simulink model "SizeDataCenterCoolingSystem"  (R2025b)
settings: Solver=daessc  StartTime=0.0  StopTime=31449600% hours ~ 8736  MaxStep=3600  RelTol=1e-3  AbsTol=1e-3
PreLoadFcn:
  | if ~exist("modelData")
  |     defaultGeographicalCoordinates;
  | end
undefined symbols (not defined in the file or in its folder): day, DiscIntNeverNeededParam, hour, modelData, month, value, year
libraries: fl_lib x63, nesl_utility x14, buildingEnergy_lib x13, datacenter_lib x5, simulink_extras x3, slpidlib x1
(part 1 of 2)
Description:
  | Data Center Cooling System Design and PUE Analysis
settings Model: Creator=vikrants  LastModifiedBy=vikrants
settings SolverCC: AutoScaleAbsTol=off  AlgebraicLoopSolver=TrustRegion  MaxZcPerStep=1.0
settings DataIOCC: SaveOutput=off  DSMLogging=off  SaveTime=off  ReturnWorkspaceOutputs=off  SignalLoggingName=logsout_SizeDataCenterCoolingSystem
settings DebuggingCC: UnconnectedInputMsg=warning  UnconnectedOutputMsg=warning  UnconnectedLineMsg=warning  SymbolicDimsDataTypeCodeGenerationDiagnostic=none
settings ModelReferenceCC: EnableRefExpFcnMdlSchedulingChecks=on
settings SFSimCC: CustomCodeUndefinedFunction=UseInterfaceOnly
settings RTWCC: GPUComputeCapability=3.5  DLArmComputeVersion=19.05
settings SimscapeCC: SimscapeLogName=simlog_DataCenterEnergyRequirement  SimscapeLogLimitData=off  SimscapeLogDataHistory=10000.0  SimscapeCompileArtifactsDiskCache=on

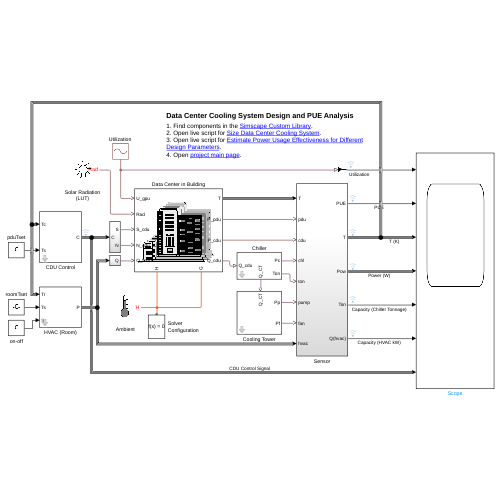
[thumbnail: Simulink's stored preview of the top-level diagram]
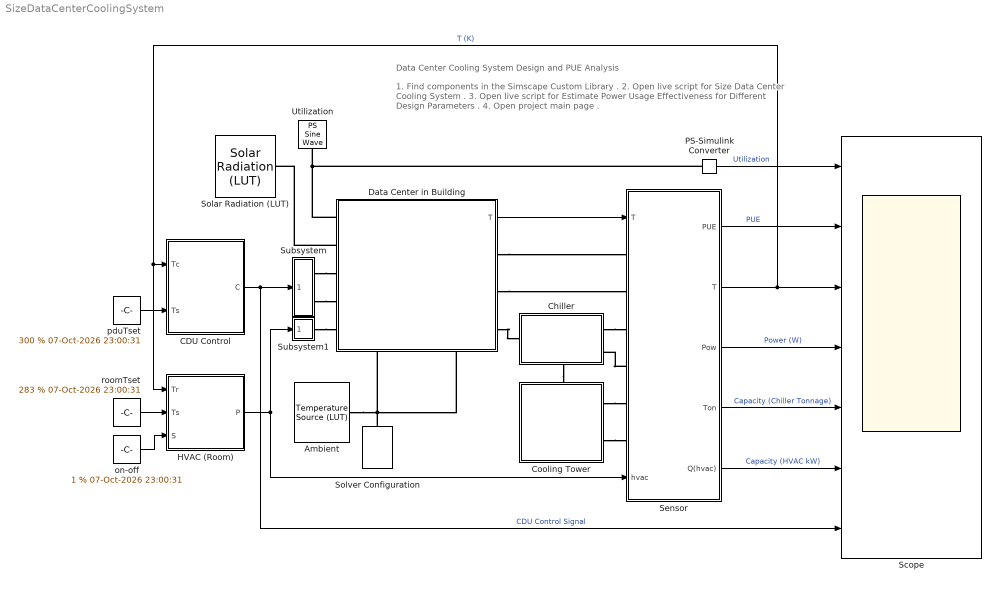
== system SizeDataCenterCoolingSystem ==
  note: 1. Find components in the Simscape Custom Library .
      | 2. Open live script for Size Data Center Cooling System .
      | 3. Open live script for Estimate Power Usage Effectiveness for Different Design Parameters .
      | 4. Open project main page .
  note: Data Center Cooling System Design and PUE Analysis
  Ambient : buildingEnergy_lib/Temperature Source (LUT)  latitude=modelData.Place.Latitude  longitude=modelData.Place.Longitude  localTime=modelData.Place.Meredian  dayLightS=0  startYear=year(modelData.StartDate)  startMonth=month(modelData.StartDate)  startDay=day(modelData.StartDate)  startHr=hour(modelData.StartDate)  numDaysData=ceil(length(modelData.DateTimeVec)/24)  interp_method=simscape.enum.interpolation.linear  extrap_method=simscape.enum.extrapolation.nearest  avgDayTvec="value(modelData.AvgDayT,\"K\") K"  pcDayTvar=modelData.AvgDayTvar  avgNightTvec="value(modelData.AvgNightT,\"K\") K"  pcNightTvar=modelData.AvgNightTvar
      settings: InternalSimscapePortConfiguration="{\"Bottom\":[],\"Left\":[],\"Right\":[{\"id\":\"H\",\"label\":\"H\",\"type\":\"foundation.thermal.thermal\"}],\"Top\":[]}"
  CDU Control : Subsystem  mask{deltaK=50, nPumps=2, tLag=1, motorSpeed=0.01, pidP=100, pidI=10, pidD=1}
      mask prompts: deltaK "Temperature window for no pumping (K)"; nPumps "Number of CDU pumps (-)"; tLag "Measurement time lag (s)"; motorSpeed "Minimum speed ratio of pump motor, 0-1 (-)"; pidP "PID controller P value"; pidI "PID controller I value"; pidD "PID controller D value"
      mask DialogControl Container2 Prompt: Measurements
      mask DialogControl Container3 Prompt: Control
  Chiller : Subsystem  mask{COP=4 % 07-Oct-2026 23:00:31}
      mask prompts: COP "COP (-)"
      settings: PortSchema="{\"entries\":[{\"content\":{\"sides\":[{\"content\":{\"connectorIds\":[\"LConn1\"]},\"type\":\"ConnectorPlacement.EquallySpacedRectSide\",\"uuid\":\"7a9d3cbb-7ec7-4e9b-b3ea-286c7e3ae193\"},{\"content\":{\"connectorIds\":[\"RConn1\",\"RConn2\"],\"side\":\"RIGHT\"},\"type\":\"ConnectorPlacement.EquallySpacedRectSide\",\"uuid\":\"cbc58f31-b5f2-4c0a-b506-28ee5b0234c2\"},{\"content\":{\"side\":\"TOP\"},\"type\":\"ConnectorPlacement.EquallySpacedRectSide\",\"uuid\":\"952b37a4-b854-4a7b-ada4-56afc544f2f3\"},{\"content\":{\"connectorIds\":[\"RConn3\"],\"side\":\"BOTTOM\"},\"type\":\"ConnectorPlacement.EquallySpacedRectSide\",\"uuid\":\"8b8e3134-7703-4e08-8e7e-92d58577d9f6\"}]},\"type\":\"ConnectorPlacement.EquallySpacedConnector\",\"uuid\":\"7e6274f1-c7d7-4742-a570-a83c5958005a\"}],\"packageUris\":[\"http://schema.mathworks.com/mf0/Connector/R2020b\"],\"version\":\"1.0\"}"
      mask DialogControl Container2 Prompt: Chiller Specifications
  Cooling Tower : Subsystem  mask{pumpHead=50, pumpEff=80 % 07-Oct-2026 23:00:31, twrFanRatio=0.02 % 07-Oct-2026 23:00:31, twrRangeDT=8 % 07-Oct-2026 23:00:31}
      mask prompts: pumpHead "Pump nominal head (m)"; pumpEff "Efficiency (%)"; twrFanRatio "Tower fan power ratio (-)"; twrRangeDT "Tower temperature range (degC)"
      settings: PortSchema="{\"entries\":[{\"content\":{\"sides\":[{\"content\":{},\"type\":\"ConnectorPlacement.EquallySpacedRectSide\",\"uuid\":\"457aae9f-8f1f-47f0-962c-a70f6cd1f469\"},{\"content\":{\"connectorIds\":[\"RConn1\",\"RConn2\"],\"side\":\"RIGHT\"},\"type\":\"ConnectorPlacement.EquallySpacedRectSide\",\"uuid\":\"5bf1e4a2-0663-4efc-92dd-183324f83000\"},{\"content\":{\"connectorIds\":[\"LConn1\"],\"side\":\"TOP\"},\"type\":\"ConnectorPlacement.EquallySpacedRectSide\",\"uuid\":\"d9f2a691-48b9-4171-b6ac-f2f0a72efb10\"}]},\"type\":\"ConnectorPlacement.EquallySpacedConnector\",\"uuid\":\"2c0f61f0-4d62-4861-80e7-d1979f22a216\"}],\"packageUris\":[\"http://schema.mathworks.com/mf0/Connector/R2020b\"],\"version\":\"1.0\"}"
      mask DialogControl Container2 Prompt: Pump
      mask DialogControl Container3 Prompt: Cooling Tower
  Data Center in Building : Subsystem
      settings: PortSchema="{\"entries\":[{\"content\":{\"sides\":[{\"content\":{\"connectorIds\":[\"LConn1\",\"LConn2\",\"LConn3\",\"LConn4\",\"LConn5\"]},\"type\":\"ConnectorPlacement.EquallySpacedRectSide\",\"uuid\":\"bcc62a9a-507d-448c-9844-f501869a29d6\"},{\"content\":{\"connectorIds\":[\"Out1\",\"RConn1\",\"RConn2\",\"RConn3\"],\"side\":\"RIGHT\"},\"type\":\"ConnectorPlacement.EquallySpacedRectSide\",\"uuid\":\"b7eb240b-2350-4e54-8431-6517b7627c9e\"},{\"content\":{\"side\":\"TOP\"},\"type\":\"ConnectorPlacement.EquallySpacedRectSide\",\"uuid\":\"331ce5d5-58db-415f-985d-83ca136d8ad7\"},{\"content\":{\"connectorIds\":[\"RConn4\",\"RConn5\"],\"side\":\"BOTTOM\"},\"type\":\"ConnectorPlacement.EquallySpacedRectSide\",\"uuid\":\"0b365461-c329-434a-a979-456a33a1343a\"}]},\"type\":\"ConnectorPlacement.EquallySpacedConnector\",\"uuid\":\"6bcf5050-5add-4254-8764-d57ae143c511\"}],\"packageUris\":[\"http://schema.mathworks.com/mf0/Connector/R2020b\"],\"version\":\"1.0\"}"
      mask Display: image('datacenterLibIcon.png');
  HVAC (Room) : Subsystem  mask{effHeatExchanger=78 % 07-Oct-2026 23:00:31, tLag=1, roomLen=100 % 07-Oct-2026 23:00:31, roomWid=40 % 07-Oct-2026 23:00:31, roomHt=5 % 07-Oct-2026 23:00:31, fracRoomVolDC=0.8 % 07-Oct-2026 23:00:31}
      mask prompts: effHeatExchanger "Efficiency (%)"; tLag "Measurement delay (s)"; roomLen "Length (m)"; roomWid "Width (m)"; roomHt "Height (m)"; fracRoomVolDC "Fraction of room volume occupied by data center (-)"
      mask DialogControl Container3 Prompt: Heat Exchanger
      mask DialogControl Container2 Prompt: Room Details
  PS-Simulink Converter : nesl_utility/PS-Simulink Converter  PhysicalDomain=network_engine_domain  SubClassName=ps_output  LeftPortType=input  RightPortType=output  PseudoPeriodic=off  Frequencies=[]  VectorFormat=inherit  Unit=inherit  AffineConversion=off
  Scope : Scope  NumInputPorts=7
      settings: ActiveDisplayYMinimum=-0.11249999999999996  ActiveDisplayYMaximum=1.1125
  Sensor : Subsystem
      settings: PortSchema="{\"entries\":[{\"content\":{\"sides\":[{\"content\":{\"connectorIds\":[\"In1\",\"LConn1\",\"LConn2\",\"LConn3\",\"LConn4\",\"LConn5\",\"LConn6\",\"In2\"]},\"type\":\"ConnectorPlacement.EquallySpacedRectSide\",\"uuid\":\"a061da3e-4dcb-442c-95d1-d8c22b8cd076\"},{\"content\":{\"connectorIds\":[\"Out1\",\"Out2\",\"Out3\",\"Out4\",\"Out5\"],\"side\":\"RIGHT\"},\"type\":\"ConnectorPlacement.EquallySpacedRectSide\",\"uuid\":\"75789351-eb15-4dd2-bcd9-a36837e8a369\"},{\"content\":{\"side\":\"TOP\"},\"type\":\"ConnectorPlacement.EquallySpacedRectSide\",\"uuid\":\"b44a6c1f-0834-4c10-bb60-11c6d0c33333\"}]},\"type\":\"ConnectorPlacement.EquallySpacedConnector\",\"uuid\":\"93d25954-c986-44d7-8262-0f4550789bd8\"}],\"packageUris\":[\"http://schema.mathworks.com/mf0/Connector/R2020b\"],\"version\":\"1.0\"}"
  Solar Radiation (LUT) : buildingEnergy_lib/Solar Radiation (LUT)  latitude=modelData.Place.Latitude  longitude=modelData.Place.Longitude  localTime=modelData.Place.Meredian  dayLightS=0  startYear=year(modelData.StartDate)  startMonth=month(modelData.StartDate)  startDay=day(modelData.StartDate)  startHr=hour(modelData.StartDate)  numHrsData=length(modelData.DateTimeVec)  cloudData=cloudCoverLibOption.none  cloudCoverVal=zeros(1, 24)  interp_method=simscape.enum.interpolation.linear  extrap_method=simscape.enum.extrapolation.nearest
      settings: InternalSimscapePortConfiguration="{\"Bottom\":[],\"Left\":[],\"Right\":[{\"id\":\"S\",\"label\":\"Rad\",\"type\":\"output\"}],\"Top\":[]}"
  Solver Configuration : nesl_utility/Solver Configuration  PhysicalDomain=network_engine_domain  SubClassName=solver  LeftPortType=input  RightPortType=generic  Tones=[]  Harmonics=[]  SimulateNoise=off  Profile=off  UseLocalSampling=off  EnableSwitchedLinearOptims=on  FrequencyDomain=off  UseCCode=off  RelTol=0.001  AbsTol=1e-06  MinStep=1e-09  ToWorkspace=off  RevertToSquareIcSolve=off  NumHomotopyIterations=100  PhasorMode=off  PhasorModeNumHarmonics=1  ConsistencySolver=NEWTON_XTOL_AFTER_FTOL  IndexReductionMethod=DerivativeReplacement  DoDC=off  ResidualTolerance=1e-09  ConsistencyTolSource=GLOBAL  ConsistencyAbsTol=0.001  ConsistencyRelTol=0.001  ConsistencyTolFactor=0.001  UseLocalSolver=off  LocalSolverChoice=NE_BACKWARD_EULER_ADVANCER  ResolveIndetEquations=on  FunctionEvalNumThread=1  LocalSolverSampleTime=0.001  DoFixedCost=off  MaxNonlinIter=3  MaxModeIter=2  ComputeImpulses=off  ImpulseIterations=2  LinearAlgebra=auto  LinearAlgebraNumThread=0  EquationFormulation=NE_TIME_EF  DelaysMemoryBudget=1024  AutomaticFiltering=on  FilteringTimeConstant=0.001  PartitionStorageMethod=AS_NEEDED  PartitionMemoryBudget=1024  PartitionMethod=ROBUST  MultibodyUseLocalSolver=off  MultibodyLocalSolverChoice=ODE1  MultibodyLocalSolverSampleTime=0.001
  Subsystem : Subsystem
  Subsystem1 : Subsystem
  Utilization : fl_lib/Physical Signals/Sources/PS Sine Wave  amplitude=0.49  bias=0.5  frequency_spec=foundation.enum.frequencySpec.frequencySI  frequency_SI=1/(4*3600) Hz  frequency_angular=1 rad/s  phase=0 rad
      settings: InternalSimscapePortConfiguration="{\"Bottom\":[],\"Left\":[],\"Right\":[{\"id\":\"O\",\"label\":\"\",\"type\":\"output\"}],\"Top\":[]}"
  on-off : Constant  Value=1 % 07-Oct-2026 23:00:31
  pduTset : Constant  Value=300 % 07-Oct-2026 23:00:31
  roomTset : Constant  Value=283 % 07-Oct-2026 23:00:31
  wires:
  Data Center in Building/1(T) -> Sensor/1("T ")
  HVAC (Room)/1(P) -> Subsystem1/1(" "), Sensor/2(hvac)
  Sensor/1(PUE) -> Scope/2  "PUE"
  Sensor/3(Pow) -> Scope/4  "Power (W)"
  Sensor/2(T) -> HVAC (Room)/1(Tr), CDU Control/1("Tc "), Scope/3  "T (K)"
  Sensor/4(Ton) -> Scope/5  "Capacity (Chiller Tonnage)"
  PS-Simulink Converter/1 -> Scope/1  "Utilization"
  CDU Control/1(C) -> Scope/7, Subsystem/1(C)  "CDU Control Signal"
  Sensor/5(Q(hvac)) -> Scope/6  "Capacity (HVAC kW)"
  roomTset/1 -> HVAC (Room)/2(Ts)
  pduTset/1 -> CDU Control/2("Ts ")
  on-off/1 -> HVAC (Room)/3(S)
  connections:
  Chiller/RConn1 -- Sensor/LConn3
  Sensor/LConn4 -- Chiller/RConn2
  Ambient/RConn1 -- Data Center in Building/RConn4 -- Data Center in Building/RConn5 -- Solver Configuration/RConn1
  PS-Simulink Converter/LConn1 -- Data Center in Building/LConn1 -- Utilization/RConn1
  Data Center in Building/RConn1 -- Sensor/LConn1
  Data Center in Building/RConn2 -- Sensor/LConn2
  Data Center in Building/RConn3 -- Chiller/LConn1
  Data Center in Building/LConn2 -- Solar Radiation (LUT)/RConn1
  Chiller/RConn3 -- Cooling Tower/LConn1
  Cooling Tower/RConn1 -- Sensor/LConn5
  Cooling Tower/RConn2 -- Sensor/LConn6
  Subsystem/RConn1 -- Data Center in Building/LConn3
  Subsystem/RConn2 -- Data Center in Building/LConn4
  Subsystem1/RConn1 -- Data Center in Building/LConn5

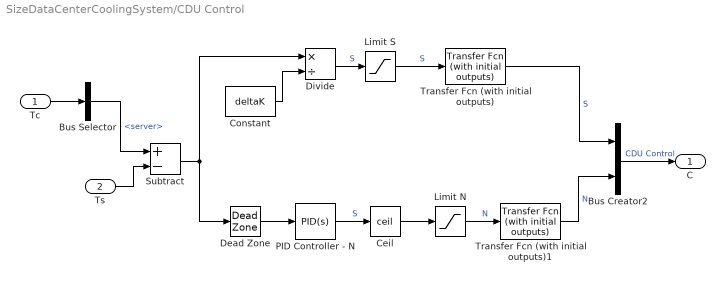
== system SizeDataCenterCoolingSystem/CDU Control ==
  "Tc " : Inport
  "Ts " : Inport  Port=2
  Bus Creator2 : BusCreator  Inputs=2
  Bus Selector : BusSelector  OutputSignals=server
  Ceil : Rounding  Operator=ceil
  Constant : Constant  Value=deltaK
  Dead Zone : DeadZone  LowerValue=-deltaK/2  UpperValue=deltaK/2  ZeroCross=off
  Divide : Product  Inputs=*/
  Limit N : Saturate  UpperLimit=nPumps  LowerLimit=0  ZeroCross=off
  Limit S : Saturate  UpperLimit=1  LowerLimit=motorSpeed  ZeroCross=off
  PID Controller - N : slpidlib/PID Controller  Controller=PID  Form=Parallel  TimeDomain=Continuous-time  UseExternalTs=off  SampleTime=-1  IntegratorMethod=Forward Euler  FilterMethod=Forward Euler  ControllerParametersSource=internal  P=pidP  I=pidI  UseKiTs=off  D=pidD  UseExternalDerivativeSource=off  N=100  UseFilter=on  TunerSelectOption=Transfer Function Based (PID Tuner App)  ZeroCross=off  InitialConditionSource=internal  InitialConditionForIntegrator=1  InitialConditionForFilter=1  DifferentiatorICPrevScaledInput=0  ExternalReset=none  TrackingMode=off  Kt=1  LimitOutput=on  SatLimitsSource=internal  UpperSaturationLimit=nPumps  LowerSaturationLimit=0  LinearizeAsGain=on  AntiWindupMode=none  Kb=1  LimitIntegrator=off  UpperIntegratorSaturationLimit=inf  LowerIntegratorSaturationLimit=-inf  POutMin=[]  POutMax=[]  IOutMin=[]  IOutMax=[]  DOutMin=[]  DOutMax=[]  NOutMin=[]  NOutMax=[]  SumOutMin=[]  SumOutMax=[]  SaturationOutMin=[]  SaturationOutMax=[]  PParamMin=[]  PParamMax=[]  IParamMin=[]  IParamMax=[]  DParamMin=[]  DParamMax=[]  NParamMin=[]  NParamMax=[]  KbParamMin=[]  KbParamMax=[]  KtParamMin=[]  KtParamMax=[]  KbOutMin=[]  KbOutMax=[]  KtOutMin=[]  KtOutMax=[]  IntegratorOutMin=[]  IntegratorOutMax=[]  FilterOutMin=[]  FilterOutMax=[]  SumI1OutMin=[]  SumI1OutMax=[]  SumI2OutMin=[]  SumI2OutMax=[]  SumI3OutMin=[]  SumI3OutMax=[]  SumI4OutMin=[]  SumI4OutMax=[]  SumDOutMin=[]  SumDOutMax=[]  DifferentiatorOutMin=[]  DifferentiatorOutMax=[]  FilterDiffOutCoefMin=[]  FilterDiffOutCoefMax=[]  ReciprocalOutMin=[]  ReciprocalOutMax=[]  SumDenOutMin=[]  SumDenOutMax=[]  SumNumOutMin=[]  SumNumOutMax=[]  DivideOutMin=[]  DivideOutMax=[]  UdiffTsProdOutMin=[]  UdiffTsProdOutMax=[]  NTsProdOutMin=[]  NTsProdOutMax=[]  UintegralTsProdOutMin=[]  UintegralTsProdOutMax=[]  UngainTsProdOutMin=[]  UngainTsProdOutMax=[]  ClampingZeroOutDataTypeStr=Inherit: Inherit via back propagation  ClampingZeroOutMin=[]  ClampingZeroOutMax=[]  FilterDenConstantOutDataTypeStr=Inherit: Inherit via back propagation  FilterDenConstantOutMin=[]  FilterDenConstantOutMax=[]  PCopyOutDataTypeStr=Inherit: Inherit via back propagation  PCopyOutMin=[]  PCopyOutMax=[]  NCopyOutDataTypeStr=Inherit: Inherit via back propagation  NCopyOutMin=[]  NCopyOutMax=[]  IntegratorContinuousStateAttributes=''  IntegratorStateMustResolveToSignalObject=off  IntegratorRTWStateStorageClass=Auto  FilterContinuousStateAttributes=''  FilterStateMustResolveToSignalObject=off  FilterRTWStateStorageClass=Auto  ParallelPVariant=InternalParameters  IdealPVariant=Disabled  IVariant=InternalParameters  DVariant=InternalParameters  IntegratorVariant=Continuous  SatVariant=Enabled  AWVariant=Passthrough  PCopyVariant=Disabled  TRVariant=Disabled  FdbkBlocksVariant=Forward  IdealPFdbkVariant=Disabled  SatFdbkVariant=Disabled  DerivativeFilterVariant=ContFilter  NVariant=InternalParameters  NCopyVariant=Disabled  FilterICVariant=InternalICsFilter  IntegratorICVariant=InternalICs  ExternalResetVariant=Disabled  TRSumVariant=Passthrough  SumFdbkVariant=Disabled  SumVariant=Sum_PID  TsampFilterVariant=InternalTs  TsampNgainVariant=Passthrough  TsampIntegralVariant=Disabled_SignalSpec  ExternalSaturationOutDataTypeStr=Inherit: Same as second input  DerivativeSourceVariant=ErrorSignal  PreIntVariant=InternalPreInt
  Subtract : Sum  Inputs=+-
  Transfer Fcn (with initial outputs) : simulink_extras/Additional Linear/Transfer Fcn (with initial outputs)  N=[1]  D="[1  tLag]"  Y0=1  U0=0
  Transfer Fcn (with initial outputs)1 : simulink_extras/Additional Linear/Transfer Fcn (with initial outputs)  N=[1]  D="[1  tLag]"  Y0=1  U0=0
  C : Outport
  wires:
  Ceil/1 -> Limit N/1
  Bus Creator2/1 -> C/1  "CDU Control"
  Dead Zone/1 -> PID Controller - N/1
  Subtract/1 -> Dead Zone/1, Divide/1
  Constant/1 -> Divide/2
  PID Controller - N/1 -> Ceil/1  "S"
  Limit N/1 -> Transfer Fcn (with initial outputs)1/1  "N"
  Divide/1 -> Limit S/1  "S"
  Limit S/1 -> Transfer Fcn (with initial outputs)/1  "S"
  "Ts "/1 -> Subtract/2
  "Tc "/1 -> Bus Selector/1
  Bus Selector/1 -> Subtract/1  "<server>"
  Transfer Fcn (with initial outputs)/1 -> Bus Creator2/1  "S"
  Transfer Fcn (with initial outputs)1/1 -> Bus Creator2/2  "N"

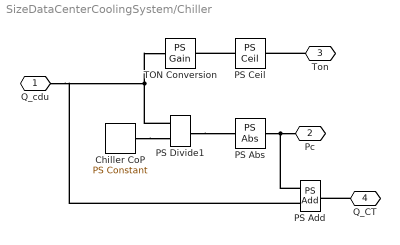
== system SizeDataCenterCoolingSystem/Chiller ==
  Chiller CoP : fl_lib/Physical Signals/Sources/PS Constant  constant=COP
  PS Abs : fl_lib/Physical Signals/Nonlinear Operators/PS Abs  ZeroCross=true
      settings: InternalSimscapePortConfiguration="{\"Bottom\":[],\"Left\":[{\"id\":\"I\",\"label\":\"\",\"type\":\"input\"}],\"Right\":[{\"id\":\"O\",\"label\":\"\",\"type\":\"output\"}],\"Top\":[]}"
  PS Add : fl_lib/Physical Signals/Functions/PS Add
  PS Ceil : fl_lib/Physical Signals/Nonlinear Operators/PS Ceil
      settings: InternalSimscapePortConfiguration="{\"Bottom\":[],\"Left\":[{\"id\":\"I\",\"label\":\"\",\"type\":\"input\"}],\"Right\":[{\"id\":\"O\",\"label\":\"\",\"type\":\"output\"}],\"Top\":[]}"
  PS Divide1 : fl_lib/Physical Signals/Functions/PS Divide
  TON Conversion : fl_lib/Physical Signals/Functions/PS Gain  gain=1/(1000*3.517) 1/W
  Q_cdu : PMIOPort  Side=Left
  Pc : PMIOPort  Port=2  Side=Right
  Ton : PMIOPort  Port=3  Side=Right
  Q_CT : PMIOPort  Port=4  Side=Right
  connections:
  PS Abs/RConn1 -- PS Add/LConn1 -- Pc/RConn1
  PS Divide1/RConn1 -- PS Abs/LConn1
  Chiller CoP/RConn1 -- PS Divide1/LConn2
  PS Ceil/LConn1 -- TON Conversion/RConn1
  PS Divide1/LConn1 -- Q_cdu/RConn1 -- PS Add/LConn2 -- TON Conversion/LConn1
  Ton/RConn1 -- PS Ceil/RConn1
  Q_CT/RConn1 -- PS Add/RConn1

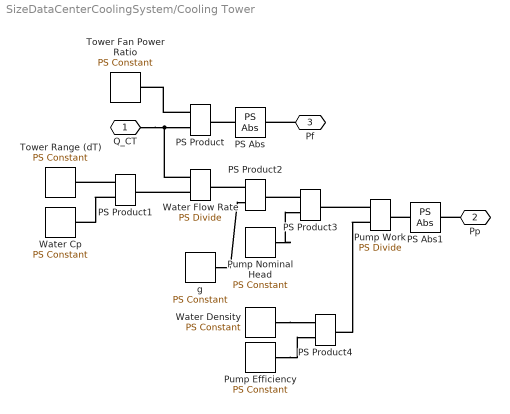
== system SizeDataCenterCoolingSystem/Cooling Tower ==
  PS Abs : fl_lib/Physical Signals/Nonlinear Operators/PS Abs  ZeroCross=true
      settings: InternalSimscapePortConfiguration="{\"Bottom\":[],\"Left\":[{\"id\":\"I\",\"label\":\"\",\"type\":\"input\"}],\"Right\":[{\"id\":\"O\",\"label\":\"\",\"type\":\"output\"}],\"Top\":[]}"
  PS Abs1 : fl_lib/Physical Signals/Nonlinear Operators/PS Abs  ZeroCross=true
      settings: InternalSimscapePortConfiguration="{\"Bottom\":[],\"Left\":[{\"id\":\"I\",\"label\":\"\",\"type\":\"input\"}],\"Right\":[{\"id\":\"O\",\"label\":\"\",\"type\":\"output\"}],\"Top\":[]}"
  PS Product{,1..4} (5 alike) : fl_lib/Physical Signals/Functions/PS Product
  Pump Efficiency : fl_lib/Physical Signals/Sources/PS Constant  constant=pumpEff/100
  Pump Nominal Head : fl_lib/Physical Signals/Sources/PS Constant  constant=pumpHead m
  Pump Work : fl_lib/Physical Signals/Functions/PS Divide
  Tower Fan Power Ratio : fl_lib/Physical Signals/Sources/PS Constant  constant=twrFanRatio
  Tower Range (dT) : fl_lib/Physical Signals/Sources/PS Constant  constant=twrRangeDT K
  Water Flow Rate : fl_lib/Physical Signals/Functions/PS Divide
  Water Cp : fl_lib/Physical Signals/Sources/PS Constant  constant=4148 J/(kg*K)
  Water Density : fl_lib/Physical Signals/Sources/PS Constant  constant=1000 kg/m^3
  g : fl_lib/Physical Signals/Sources/PS Constant  constant=9.81 m/s^2
  Q_CT : PMIOPort  Side=Left
  Pp : PMIOPort  Port=2  Side=Right
  Pf : PMIOPort  Port=3  Side=Right
  connections:
  PS Abs/LConn1 -- PS Product/RConn1
  PS Product1/LConn2 -- Water Cp/RConn1
  PS Product1/LConn1 -- Tower Range (dT)/RConn1
  Water Flow Rate/LConn2 -- PS Product1/RConn1
  PS Product/LConn1 -- Tower Fan Power Ratio/RConn1
  Q_CT/RConn1 -- Water Flow Rate/LConn1 -- PS Product/LConn2
  PS Product2/LConn1 -- Water Flow Rate/RConn1
  g/RConn1 -- PS Product2/LConn2
  PS Product3/LConn1 -- PS Product2/RConn1
  Pump Nominal Head/RConn1 -- PS Product3/LConn2
  Water Density/RConn1 -- PS Product4/LConn1
  Pump Efficiency/RConn1 -- PS Product4/LConn2
  Pump Work/LConn1 -- PS Product3/RConn1
  Pump Work/LConn2 -- PS Product4/RConn1
  PS Abs1/LConn1 -- Pump Work/RConn1
  Pf/RConn1 -- PS Abs/RConn1
  Pp/RConn1 -- PS Abs1/RConn1

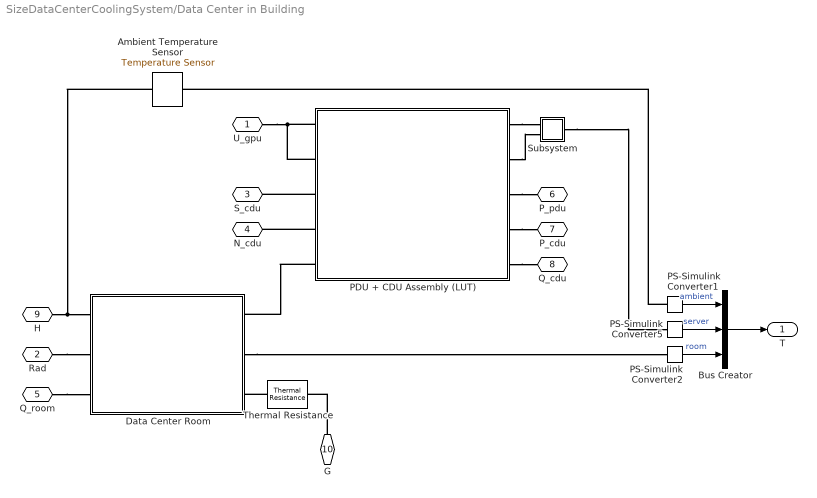
== system SizeDataCenterCoolingSystem/Data Center in Building ==
  Ambient Temperature Sensor : fl_lib/Thermal/Thermal Sensors/Temperature Sensor  temperature_measure=foundation.enum.MeasurementReference.absolute
      settings: InternalSimscapePortConfiguration="{\"Bottom\":[],\"Left\":[{\"id\":\"A\",\"label\":\"A\",\"type\":\"foundation.thermal.thermal\"}],\"Right\":[{\"id\":\"T\",\"label\":\"T\",\"type\":\"output\"}],\"Top\":[]}"
  Bus Creator : BusCreator  Inputs=3
  Data Center Room : Subsystem  mask{roomLength=100 % 07-Oct-2026 23:00:31, roomWidth=40 % 07-Oct-2026 23:00:31, roomHeight=5 % 07-Oct-2026 23:00:31, rotateDeg=30 % 07-Oct-2026 23:00:31, wallAngle=90, wallThickness=0.1 % 07-Oct-2026 23:00:31, roofThickness=0.08 % 07-Oct-2026 23:00:31, floorThickness=0.11 % 07-Oct-2026 23:00:31, glassThickness=0.005 % 07-Oct-2026 23:00:31, fracDCvol=0.8 % 07-Oct-2026 23:00:31, windowFracWall1=0.75 % 07-Oct-2026 23:00:31, windowFracWall2=0.01 % 07-Oct-2026 23:00:31, windowFracWall3=0.75 % 07-Oct-2026 23:00:31, windowFracWall4=0.01 % 07-Oct-2026 23:00:31, wallDensity=4000, wallCp=1870, wallThermalK=2, wallAbsorptivity=0.5, glassDensity=2500, glassCp=787, glassThermalK=1, glassAbsorptivity=0.35, glassTransmissivity=0.45 % 07-Oct-2026 23:00:31, initialTemp=value(modelData.AvgDayT(1,1),"K"), htcExternal=50, htcInternal=10, latitude=modelData.Place.Latitude, longitude=modelData.Place.Longitude, meredian=modelData.Place.Meredian, dayLightSaving=0, year=year(modelData.StartDate), month=month(modelData.StartDate), day=day(modelData.StartDate), hour=hour(modelData.StartDate), totalHours=length(modelData.DateTimeVec)}
      mask prompts: roomLength "Length (m)"; roomWidth "Width (m)"; roomHeight "Height (m)"; rotateDeg "Room orientation wrt South (deg)"; wallAngle "Wall angle wrt ground (deg)"; wallThickness "Room wall thickness (m)"; roofThickness "Room roof thickness (m)"; floorThickness "Room floor thickness (m)"; glassThickness "Window glass thickness (m)"; fracDCvol "Fraction room volume occupied by Data Center units (-)"; windowFracWall1 "Fraction wall 1 area occupied by window (-)"; windowFracWall2 "Fraction wall 2 area occupied by window (-)"; windowFracWall3 "Fraction wall 3 area occupied by window (-)"; windowFracWall4 "Fraction wall 4 area occupied by window (-)"; wallDensity "Density (kg/m^3)"; wallCp "Heat capacity (J/kg*K)"; wallThermalK "Thermal conductivity (W/K*m)"; wallAbsorptivity "Solar absorptivity (-)"; glassDensity "Density (kg/m^3)"; glassCp "Heat capacity (J/Kg*K)"; glassThermalK "Thermal conductivity (W/K*m)"; glassAbsorptivity "Solar absorptivity (-)"; glassTransmissivity "Solar transmissivity (-)"; initialTemp "Initial temperature (K)"; htcExternal "Heat transfer coefficient from ambient to walls (W/K*m^2)"; htcInternal "Heat transfer coefficient from room air to walls (W/K*m^2)"; latitude "Latitude (deg)"; longitude "Longitude (deg)"; meredian "Longitude reference for local time (deg)"; dayLightSaving "Day light saving hours (hrs)"; year "Start time year (-)"; month "Start time month (-)"; day "Start time day (-)"; hour "Start time hour of the day (-)"; totalHours "Total hours of timeseries (-)"
      mask DialogControl RoomDimensionSpec Prompt: Room Dimension
      mask DialogControl WallMaterialProp Prompt: Wall Material
      mask DialogControl WindowGlassMatProp Prompt: Window Glass Material
      mask DialogControl HeatTransferParam Prompt: Heat Transfer
      mask DialogControl LocationAndTime Prompt: Location and Timeframe
  PDU + CDU Assembly (LUT) : Subsystem  mask{nAssembly=36, nRacks=3, nTrays=6, flowrate_vec=[0.3, 0.5, 1.0, 1.3, 1.7, 2, 2.6, 3.3, 3.5, 3.7]/998, capacity_vec=[3,9,36,60,104,144,243,392,441,492]*1000, numPump=2, effPump_vec=[0.4,0.42,0.45,0.5,0.55,0.6,0.62,0.65,0.65,0.64], prDrop_mat=100000*[0.28,1.1,2.5,4,5.2,8,13,18.5,23,27.78; 0.56,2.22,5,7.8,12,16.5,25,37,45,55.56]', speed=2, trayMass=5, trayCp=2000, trayThermalR=0.1, nGPU=1, gpuTDPperDie=1200, gpuIdlePower=300, gpuHBMpower=80, gpuExponent=1.4, gpuHBMutil=0.7, gpuLeakage=1.5, gpuNominalDieT=350, gpuDieThermalC=50, gpuHeatSinkR=1e-3, gpuSurfArea=0.01, gpuAmbientR=1e-3, nCPU=1, cpuTDPperSocket=350, cpuIdlePower=80, cpuExponent=1.1, cpuLeakage=1.5, cpuNominalDieT=350, cpuDieThermalC=50, cpuHeatSinkR=1e-3, cpuSurfArea=0.01, cpuAmbientR=1e-3, initialT=value(modelData.AvgDayT(1,1),"K"), htc=10}
      mask prompts: nAssembly "Number of PDU+CDU assemblies (-)"; nRacks "Number of racks (-)"; nTrays "Number of IT trays per rack (-)"; flowrate_vec "Coolant volumetric flowrate vector (m^3/s)"; capacity_vec "Heat exchanger capacity vector (W)"; numPump "Total number of pumps in each assembly (-)"; effPump_vec "Pump efficiency vector, 0-1 (-)"; prDrop_mat "Pressure drop (Pa)"; speed "Pump speed scaling (-)"; trayMass "Tray mass (kg)"; trayCp "Tray specific heat capacity (J/kg*K)"; trayThermalR "Tray to external thermal resistance (K/W)"; nGPU "Number of GPU per tray (-)"; gpuTDPperDie "GPU TDP per die (W)"; gpuIdlePower "GPU idle power (W)"; gpuHBMpower "HBM power per GPU (W)"; gpuExponent "GPU power utilization exponent (-)"; gpuHBMutil "HBM utilization as fraction of compute utilization (-)"; gpuLeakage "Leakage increase per K above nominal temperature (W/K)"; gpuNominalDieT "Nominal die temperature at TDP (K)"; gpuDieThermalC "GPU die thermal capacitance (J/K)"; gpuHeatSinkR "GPU die-heat-sink thermal resistance (K/W)"; gpuSurfArea "Surface area per die for ambient heat transfer (m^2)"; gpuAmbientR "GPU die-ambient thermal resistance (K/W)"; nCPU "Number of CPU per tray (-)"; cpuTDPperSocket "CPU TDP per socket (W)"; cpuIdlePower "CPU idle power per socket (W)"; cpuExponent "CPU power utilization exponent (-)"; cpuLeakage "Leakage increase per K above nominal temperature (W/K)"; cpuNominalDieT "Nominal die temperature at TDP (K)"; cpuDieThermalC "CPU die thermal capacitance (J/K)"; cpuHeatSinkR "CPU die-heat-sink thermal resistance (K/W)"; cpuSurfArea "Surface area per die for ambient heat transfer (m^2)"; cpuAmbientR "CPU die-ambient thermal resistance (K/W)"; initialT "Initial temperature (K)"; htc "Heat transfer coefficient to ambient (W/m^2.K)"
      settings: CopyFcn=set_param(gcbh,'LinkStatus','none');
      mask Help: web("DocumentationPDUCDUAssemblyLUT.html")
      mask DialogControl Container10 Prompt: PDU Racks
      mask DialogControl getRatingButton Prompt: Get Rating
      mask DialogControl Container11 Prompt: CDU
      mask DialogControl Container9 Prompt: IT Tray
      mask DialogControl Container6 Prompt: GPU
      mask DialogControl Container7 Prompt: CPU
      mask DialogControl Container8 Prompt: Initial Conditions
      mask Display: image('icon_AssemblyLUT.png');
  PS-Simulink Converter1 : nesl_utility/PS-Simulink Converter  PhysicalDomain=network_engine_domain  SubClassName=ps_output  LeftPortType=input  RightPortType=output  PseudoPeriodic=off  Frequencies=[]  VectorFormat=inherit  Unit=inherit  AffineConversion=off
  PS-Simulink Converter2 : nesl_utility/PS-Simulink Converter  PhysicalDomain=network_engine_domain  SubClassName=ps_output  LeftPortType=input  RightPortType=output  PseudoPeriodic=off  Frequencies=[]  VectorFormat=inherit  Unit=inherit  AffineConversion=off
  PS-Simulink Converter5 : nesl_utility/PS-Simulink Converter  PhysicalDomain=network_engine_domain  SubClassName=ps_output  LeftPortType=input  RightPortType=output  PseudoPeriodic=off  Frequencies=[]  VectorFormat=inherit  Unit=inherit  AffineConversion=off
  Subsystem : Subsystem
  Thermal Resistance : fl_lib/Thermal/Thermal Elements/Thermal Resistance  resistance=1 K/W  T_specify=off  T_priority=None  T=0 K  T_nominal_specify=off  T_nominal_value=1  T_nominal_unit=K  Q_specify=off  Q_priority=None  Q=0 W  Q_nominal_specify=off  Q_nominal_value=1  Q_nominal_unit=W
  U_gpu : PMIOPort  Side=Left
  Rad : PMIOPort  Port=2  Side=Left
  S_cdu : PMIOPort  Port=3  Side=Left
  N_cdu : PMIOPort  Port=4  Side=Left
  Q_room : PMIOPort  Port=5  Side=Left
  P_pdu : PMIOPort  Port=6  Side=Right
  P_cdu : PMIOPort  Port=7  Side=Right
  Q_cdu : PMIOPort  Port=8  Side=Right
  H : PMIOPort  Port=9  Side=Right
  G : PMIOPort  Port=10  Side=Right
  T : Outport
  wires:
  PS-Simulink Converter1/1 -> Bus Creator/1  "ambient"
  PS-Simulink Converter5/1 -> Bus Creator/2  "server"
  PS-Simulink Converter2/1 -> Bus Creator/3  "room"
  Bus Creator/1 -> T/1
  connections:
  PDU + CDU Assembly (LUT)/LConn3 -- S_cdu/RConn1
  PDU + CDU Assembly (LUT)/RConn2 -- Subsystem/LConn2
  U_gpu/RConn1 -- PDU + CDU Assembly (LUT)/LConn1 -- PDU + CDU Assembly (LUT)/LConn2
  PDU + CDU Assembly (LUT)/RConn4 -- P_cdu/RConn1
  PDU + CDU Assembly (LUT)/RConn5 -- Q_cdu/RConn1
  PDU + CDU Assembly (LUT)/LConn4 -- N_cdu/RConn1
  PDU + CDU Assembly (LUT)/RConn3 -- P_pdu/RConn1
  PDU + CDU Assembly (LUT)/RConn1 -- Subsystem/LConn1
  Subsystem/RConn1 -- PS-Simulink Converter5/LConn1
  H/RConn1 -- Ambient Temperature Sensor/LConn1 -- Data Center Room/LConn1
  Rad/RConn1 -- Data Center Room/LConn2
  PDU + CDU Assembly (LUT)/LConn5 -- Data Center Room/RConn1
  Data Center Room/RConn2 -- PS-Simulink Converter2/LConn1
  Q_room/RConn1 -- Data Center Room/LConn3
  Thermal Resistance/LConn1 -- Data Center Room/RConn3
  PS-Simulink Converter1/LConn1 -- Ambient Temperature Sensor/RConn1
  G/RConn1 -- Thermal Resistance/RConn1

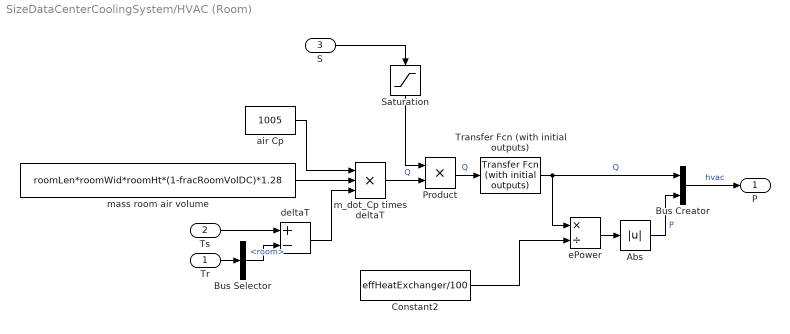
== system SizeDataCenterCoolingSystem/HVAC (Room) ==
  Tr : Inport
  Ts : Inport  Port=2
  S : Inport  Port=3
  Abs : Abs  SaturateOnIntegerOverflow=off
  Bus Creator : BusCreator  Inputs=2
  Bus Selector : BusSelector  OutputSignals=room
  Constant2 : Constant  Value=effHeatExchanger/100
  Product : Product
  Saturation : Saturate  UpperLimit=1  LowerLimit=0  ZeroCross=off
  Transfer Fcn (with initial outputs) : simulink_extras/Additional Linear/Transfer Fcn (with initial outputs)  N=[1]  D="[1  tLag]"  Y0=0  U0=0
  air Cp : Constant  Value=1005
  deltaT : Sum  Inputs=+-
  ePower : Product  Inputs=*/
  m_dot_Cp times deltaT : Product  Inputs=3
  mass room air volume : Constant  Value=roomLen*roomWid*roomHt*(1-fracRoomVolDC)*1.28
  P : Outport
  wires:
  Ts/1 -> deltaT/1
  deltaT/1 -> m_dot_Cp times deltaT/3
  Tr/1 -> Bus Selector/1
  Bus Selector/1 -> deltaT/2  "<room>"
  Constant2/1 -> ePower/2
  ePower/1 -> Abs/1
  air Cp/1 -> m_dot_Cp times deltaT/1
  mass room air volume/1 -> m_dot_Cp times deltaT/2
  Abs/1 -> Bus Creator/2  "P"
  Bus Creator/1 -> P/1  "hvac"
  S/1 -> Saturation/1
  m_dot_Cp times deltaT/1 -> Product/2  "Q"
  Product/1 -> Transfer Fcn (with initial outputs)/1  "Q"
  Saturation/1 -> Product/1
  Transfer Fcn (with initial outputs)/1 -> ePower/1, Bus Creator/1  "Q"

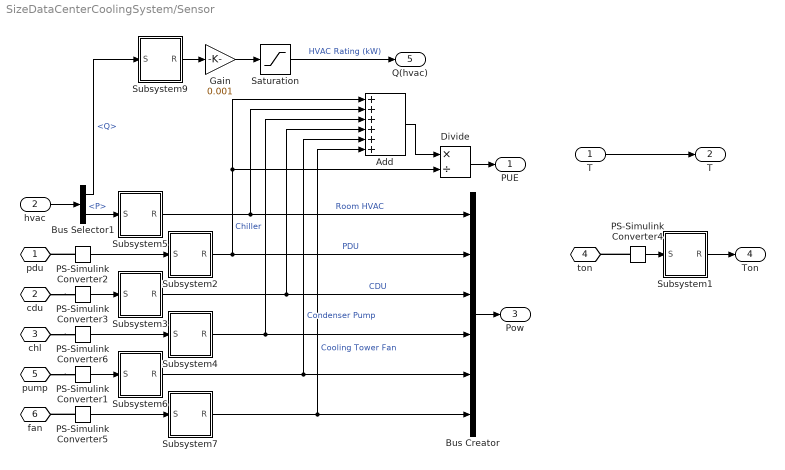
== system SizeDataCenterCoolingSystem/Sensor ==
  "T " : Inport
  hvac : Inport  Port=2
  Add : Sum  Inputs=++++++
  Bus Creator : BusCreator  Inputs=6
  Bus Selector1 : BusSelector  OutputSignals=Q,P
  Divide : Product  Inputs=*/
  Gain : Gain  Gain=0.001
  PS-Simulink Converter{1..6} (6 alike) : nesl_utility/PS-Simulink Converter  PhysicalDomain=network_engine_domain  SubClassName=ps_output  LeftPortType=input  RightPortType=output  PseudoPeriodic=off  Frequencies=[]  VectorFormat=inherit  Unit=inherit  AffineConversion=off
  Saturation : Saturate  UpperLimit=10000  LowerLimit=-10000
  Subsystem1 : Subsystem  mask{sampleTimeSec=6}
      mask prompts: sampleTimeSec "Sample time (s)"
  Subsystem2 : Subsystem  mask{sampleTimeSec=6}
      mask prompts: sampleTimeSec "Sample time (s)"
  Subsystem3 : Subsystem  mask{sampleTimeSec=6}
      mask prompts: sampleTimeSec "Sample time (s)"
  Subsystem4 : Subsystem  mask{sampleTimeSec=6}
      mask prompts: sampleTimeSec "Sample time (s)"
  Subsystem5 : Subsystem  mask{sampleTimeSec=6}
      mask prompts: sampleTimeSec "Sample time (s)"
  Subsystem6 : Subsystem  mask{sampleTimeSec=6}
      mask prompts: sampleTimeSec "Sample time (s)"
  Subsystem7 : Subsystem  mask{sampleTimeSec=6}
      mask prompts: sampleTimeSec "Sample time (s)"
  Subsystem9 : Subsystem  mask{sampleTimeSec=6}
      mask prompts: sampleTimeSec "Sample time (s)"
  pdu : PMIOPort  Side=Left
  cdu : PMIOPort  Port=2  Side=Left
  chl : PMIOPort  Port=3  Side=Left
  ton : PMIOPort  Port=4  Side=Left
  pump : PMIOPort  Port=5  Side=Left
  fan : PMIOPort  Port=6  Side=Left
  PUE : Outport
  T : Outport  Port=2
  Pow : Outport  Port=3
  Ton : Outport  Port=4
  Q(hvac) : Outport  Port=5
  wires:
  PS-Simulink Converter4/1 -> Subsystem1/1(S)
  PS-Simulink Converter3/1 -> Subsystem3/1(S)
  PS-Simulink Converter6/1 -> Subsystem4/1(S)
  Bus Creator/1 -> Pow/1
  PS-Simulink Converter2/1 -> Subsystem2/1(S)
  Subsystem1/1(R) -> Ton/1
  Subsystem2/1(R) -> Add/1, Divide/2, Bus Creator/2  "PDU"
  Subsystem3/1(R) -> Add/4, Bus Creator/3  "CDU"
  Subsystem4/1(R) -> Add/3, Bus Creator/4  "Chiller"
  "T "/1 -> T/1
  Subsystem5/1(R) -> Bus Creator/1, Add/2  "Room HVAC"
  Divide/1 -> PUE/1
  Add/1 -> Divide/1
  hvac/1 -> Bus Selector1/1
  Bus Selector1/2 -> Subsystem5/1(S)  "<P>"
  Bus Selector1/1 -> Subsystem9/1(S)  "<Q>"
  Subsystem9/1(R) -> Gain/1
  Gain/1 -> Saturation/1
  Saturation/1 -> Q(hvac)/1  "HVAC Rating (kW)"
  PS-Simulink Converter1/1 -> Subsystem6/1(S)
  PS-Simulink Converter5/1 -> Subsystem7/1(S)
  Subsystem6/1(R) -> Bus Creator/5, Add/5  "Condenser Pump"
  Subsystem7/1(R) -> Add/6, Bus Creator/6  "Cooling Tower Fan"
  connections:
  PS-Simulink Converter4/LConn1 -- ton/RConn1
  PS-Simulink Converter2/LConn1 -- pdu/RConn1
  cdu/RConn1 -- PS-Simulink Converter3/LConn1
  chl/RConn1 -- PS-Simulink Converter6/LConn1
  pump/RConn1 -- PS-Simulink Converter1/LConn1
  PS-Simulink Converter5/LConn1 -- fan/RConn1

== system SizeDataCenterCoolingSystem/Subsystem ==
  C : Inport
  Bus Selector : BusSelector  OutputSignals=S,N
  Simulink-PS Converter : nesl_utility/Simulink-PS Converter  PhysicalDomain=network_engine_domain  SubClassName=ps_input  LeftPortType=input  RightPortType=output  PseudoPeriodic=off  Frequencies=[]  NoiseDistribution=none  NoiseParameters=[]  Unit=1  AffineConversion=off  FilteringAndDerivatives=provide  SimscapeFilterOrder=1  InputFilterTimeConstant=0.001  UdotUserProvided=0
  Simulink-PS Converter1 : nesl_utility/Simulink-PS Converter  PhysicalDomain=network_engine_domain  SubClassName=ps_input  LeftPortType=input  RightPortType=output  PseudoPeriodic=off  Frequencies=[]  NoiseDistribution=none  NoiseParameters=[]  Unit=1  AffineConversion=off  FilteringAndDerivatives=provide  SimscapeFilterOrder=1  InputFilterTimeConstant=0.001  UdotUserProvided=0
  S : PMIOPort  Side=Right
  N : PMIOPort  Port=2  Side=Right
  wires:
  Bus Selector/1 -> Simulink-PS Converter/1  "<S>"
  Bus Selector/2 -> Simulink-PS Converter1/1  "<N>"
  C/1 -> Bus Selector/1
  connections:
  Simulink-PS Converter1/RConn1 -- N/RConn1
  Simulink-PS Converter/RConn1 -- S/RConn1

== system SizeDataCenterCoolingSystem/Subsystem1 ==
  " " : Inport
  Bus Selector : BusSelector  OutputSignals=Q
  Simulink-PS Converter : nesl_utility/Simulink-PS Converter  PhysicalDomain=network_engine_domain  SubClassName=ps_input  LeftPortType=input  RightPortType=output  PseudoPeriodic=off  Frequencies=[]  NoiseDistribution=none  NoiseParameters=[]  Unit=1  AffineConversion=off  FilteringAndDerivatives=provide  SimscapeFilterOrder=1  InputFilterTimeConstant=0.001  UdotUserProvided=0
  Q : PMIOPort  Side=Right
  wires:
  Bus Selector/1 -> Simulink-PS Converter/1  "<Q>"
  " "/1 -> Bus Selector/1
  connections:
  Simulink-PS Converter/RConn1 -- Q/RConn1

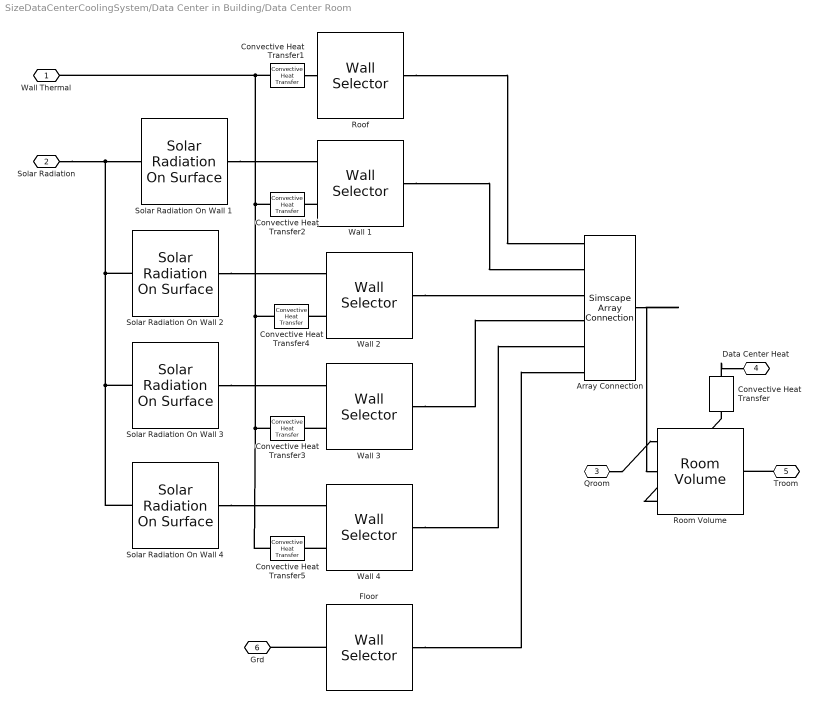
== system SizeDataCenterCoolingSystem/Data Center in Building/Data Center Room ==
  Array Connection : SimscapeArrayConnection  Domain=foundation.thermal.thermal  NumScalarElements=6
  Convective Heat Transfer : fl_lib/Thermal/Thermal Elements/Convective Heat Transfer  thermal_type=foundation.enum.constant_variable.constant  area=(2*(roomLength+roomWidth)*roomHeight+roomLength*roomWidth)*((1-fracDCvol)^(2/3)) m^2  heat_tr_coeff=htcInternal W/(K*m^2)  min_heat_tr_coeff=1e-3 W/(K*m^2)  T_specify=off  T_priority=None  T=0 K  T_nominal_specify=off  T_nominal_value=1  T_nominal_unit=K  Q_specify=off  Q_priority=None  Q=0 W  Q_nominal_specify=off  Q_nominal_value=1  Q_nominal_unit=W
  Convective Heat Transfer1 : fl_lib/Thermal/Thermal Elements/Convective Heat Transfer  thermal_type=foundation.enum.constant_variable.constant  area=roomLength*roomWidth m^2  heat_tr_coeff=htcExternal W/(K*m^2)  min_heat_tr_coeff=1e-3 W/(K*m^2)  T_specify=off  T_priority=None  T=0 K  T_nominal_specify=off  T_nominal_value=1  T_nominal_unit=K  Q_specify=off  Q_priority=None  Q=0 W  Q_nominal_specify=off  Q_nominal_value=1  Q_nominal_unit=W
  Convective Heat Transfer2 : fl_lib/Thermal/Thermal Elements/Convective Heat Transfer  thermal_type=foundation.enum.constant_variable.constant  area=roomLength*roomHeight m^2  heat_tr_coeff=htcExternal W/(K*m^2)  min_heat_tr_coeff=1e-3 W/(K*m^2)  T_specify=off  T_priority=None  T=0 K  T_nominal_specify=off  T_nominal_value=1  T_nominal_unit=K  Q_specify=off  Q_priority=None  Q=0 W  Q_nominal_specify=off  Q_nominal_value=1  Q_nominal_unit=W
  Convective Heat Transfer3 : fl_lib/Thermal/Thermal Elements/Convective Heat Transfer  thermal_type=foundation.enum.constant_variable.constant  area=roomLength*roomHeight m^2  heat_tr_coeff=htcExternal W/(K*m^2)  min_heat_tr_coeff=1e-3 W/(K*m^2)  T_specify=off  T_priority=None  T=0 K  T_nominal_specify=off  T_nominal_value=1  T_nominal_unit=K  Q_specify=off  Q_priority=None  Q=0 W  Q_nominal_specify=off  Q_nominal_value=1  Q_nominal_unit=W
  Convective Heat Transfer4 : fl_lib/Thermal/Thermal Elements/Convective Heat Transfer  thermal_type=foundation.enum.constant_variable.constant  area=roomWidth*roomHeight m^2  heat_tr_coeff=htcExternal W/(K*m^2)  min_heat_tr_coeff=1e-3 W/(K*m^2)  T_specify=off  T_priority=None  T=0 K  T_nominal_specify=off  T_nominal_value=1  T_nominal_unit=K  Q_specify=off  Q_priority=None  Q=0 W  Q_nominal_specify=off  Q_nominal_value=1  Q_nominal_unit=W
  Convective Heat Transfer5 : fl_lib/Thermal/Thermal Elements/Convective Heat Transfer  thermal_type=foundation.enum.constant_variable.constant  area=roomWidth*roomHeight m^2  heat_tr_coeff=htcExternal W/(K*m^2)  min_heat_tr_coeff=1e-3 W/(K*m^2)  T_specify=off  T_priority=None  T=0 K  T_nominal_specify=off  T_nominal_value=1  T_nominal_unit=K  Q_specify=off  Q_priority=None  Q=0 W  Q_nominal_specify=off  Q_nominal_value=1  Q_nominal_unit=W
  Floor : buildingEnergy_lib/Wall Selector  optWall=wallModelOption.wallOnly  wallLength=roomLength m  wallHeight=roomWidth m  wallThickness=floorThickness m  wallMaterialDen=wallDensity kg/m^3  wallMaterialCp=wallCp J/(K*kg)  wallAbsorptivity=0.5  wallThermalK=wallThermalK W/(K*m)  winLength=1 m  winHeight=0.5 m  winThickness=0.007 m  winMaterialDen=2500 kg/m^3  winMaterialCp=787 J/(K*kg)  winAbsorptivity=0.35  winThermalK=1 W/(K*m)  winTransmissivity=0.45  ventLength=0.1 m  ventHeight=0.1 m  extToWallHTC=htcExternal W/(K*m^2)  intToRoomHTC=htcInternal W/(K*m^2)  iniT=initialTemp K
      settings: InternalSimscapePortConfiguration="{\"Bottom\":[],\"Left\":[{\"id\":\"A\",\"label\":\"A\",\"type\":\"foundation.thermal.thermal\"}],\"Right\":[{\"id\":\"B\",\"label\":\"B\",\"type\":\"foundation.thermal.thermal\"}],\"Top\":[]}"
  Roof : buildingEnergy_lib/Wall Selector  optWall=wallModelOption.wallOnly  wallLength=roomLength m  wallHeight=roomWidth m  wallThickness=roofThickness m  wallMaterialDen=wallDensity kg/m^3  wallMaterialCp=wallCp J/(K*kg)  wallAbsorptivity=0.5  wallThermalK=wallThermalK W/(K*m)  winLength=1 m  winHeight=0.5 m  winThickness=0.007 m  winMaterialDen=2500 kg/m^3  winMaterialCp=787 J/(K*kg)  winAbsorptivity=0.35  winThermalK=1 W/(K*m)  winTransmissivity=0.45  ventLength=0.1 m  ventHeight=0.1 m  extToWallHTC=htcExternal W/(K*m^2)  intToRoomHTC=htcInternal W/(K*m^2)  iniT=initialTemp K
      settings: InternalSimscapePortConfiguration="{\"Bottom\":[],\"Left\":[{\"id\":\"A\",\"label\":\"A\",\"type\":\"foundation.thermal.thermal\"}],\"Right\":[{\"id\":\"B\",\"label\":\"B\",\"type\":\"foundation.thermal.thermal\"}],\"Top\":[]}"
  Room Volume : buildingEnergy_lib/Room Volume  N1=6  N2=1  iniT=initialTemp K  length=roomLength*(1-fracDCvol) m  width=roomWidth m  height=roomHeight m
      settings: InternalSimscapePortConfiguration="{\"Bottom\":[],\"Left\":[{\"id\":\"S\",\"label\":\"S\",\"type\":\"input\"}],\"Right\":[{\"id\":\"T\",\"label\":\"T\",\"type\":\"output\"}],\"Top\":[{\"id\":\"M1\",\"label\":\"M1\",\"type\":\"foundation.thermal.thermal\"},{\"id\":\"M2\",\"label\":\"M2\",\"type\":\"foundation.thermal.thermal\"}]}"
  Solar Radiation On Wall 1 : buildingEnergy_lib/Solar Radiation On Surface  latitude=latitude  longitude=longitude  localTime=meredian  dayLightS=dayLightSaving  surfAngle=wallAngle deg  surfUnitV=[0*cos(deg2rad(rotateDeg))-(-1)*sin(deg2rad(rotateDeg)), 0*sin(deg2rad(rotateDeg))+(-1)*cos(deg2rad(rotateDeg))]  startYear=year  startMonth=month  startDay=day  startHr=hour  numHrsData=totalHours  interp_method=simscape.enum.interpolation.linear  extrap_method=simscape.enum.extrapolation.nearest
      settings: InternalSimscapePortConfiguration="{\"Bottom\":[],\"Left\":[{\"id\":\"S\",\"label\":\"Rad\",\"type\":\"input\"}],\"Right\":[{\"id\":\"Sf\",\"label\":\"S\",\"type\":\"output\"}],\"Top\":[]}"
  Solar Radiation On Wall 2 : buildingEnergy_lib/Solar Radiation On Surface  latitude=latitude  longitude=longitude  localTime=meredian  dayLightS=dayLightSaving  surfAngle=wallAngle deg  surfUnitV=[1*cos(deg2rad(rotateDeg))-0*sin(deg2rad(rotateDeg)), 1*sin(deg2rad(rotateDeg))+0*cos(deg2rad(rotateDeg))]  startYear=year  startMonth=month  startDay=day  startHr=hour  numHrsData=totalHours  interp_method=simscape.enum.interpolation.linear  extrap_method=simscape.enum.extrapolation.nearest
      settings: InternalSimscapePortConfiguration="{\"Bottom\":[],\"Left\":[{\"id\":\"S\",\"label\":\"Rad\",\"type\":\"input\"}],\"Right\":[{\"id\":\"Sf\",\"label\":\"S\",\"type\":\"output\"}],\"Top\":[]}"
  Solar Radiation On Wall 3 : buildingEnergy_lib/Solar Radiation On Surface  latitude=latitude  longitude=longitude  localTime=meredian  dayLightS=dayLightSaving  surfAngle=wallAngle deg  surfUnitV=[0*cos(deg2rad(rotateDeg))-1*sin(deg2rad(rotateDeg)), 0*sin(deg2rad(rotateDeg))+1*cos(deg2rad(rotateDeg))]  startYear=year  startMonth=month  startDay=day  startHr=hour  numHrsData=totalHours  interp_method=simscape.enum.interpolation.linear  extrap_method=simscape.enum.extrapolation.nearest
      settings: InternalSimscapePortConfiguration="{\"Bottom\":[],\"Left\":[{\"id\":\"S\",\"label\":\"Rad\",\"type\":\"input\"}],\"Right\":[{\"id\":\"Sf\",\"label\":\"S\",\"type\":\"output\"}],\"Top\":[]}"
  Solar Radiation On Wall 4 : buildingEnergy_lib/Solar Radiation On Surface  latitude=latitude  longitude=longitude  localTime=meredian  dayLightS=dayLightSaving  surfAngle=wallAngle deg  surfUnitV=[(-1)*cos(deg2rad(rotateDeg))-0*sin(deg2rad(rotateDeg)), (-1)*sin(deg2rad(rotateDeg))+0*cos(deg2rad(rotateDeg))]  startYear=year  startMonth=month  startDay=day  startHr=hour  numHrsData=totalHours  interp_method=simscape.enum.interpolation.linear  extrap_method=simscape.enum.extrapolation.nearest
      settings: InternalSimscapePortConfiguration="{\"Bottom\":[],\"Left\":[{\"id\":\"S\",\"label\":\"Rad\",\"type\":\"input\"}],\"Right\":[{\"id\":\"Sf\",\"label\":\"S\",\"type\":\"output\"}],\"Top\":[]}"
  Wall 1 : buildingEnergy_lib/Wall Selector  optWall=wallModelOption.wallSolarWin  wallLength=roomLength m  wallHeight=roomHeight m  wallThickness=wallThickness m  wallMaterialDen=wallDensity kg/m^3  wallMaterialCp=wallCp J/(K*kg)  wallAbsorptivity=wallAbsorptivity  wallThermalK=wallThermalK W/(K*m)  winLength=roomLength*windowFracWall1 m  winHeight=roomHeight m  winThickness=glassThickness m  winMaterialDen=glassDensity kg/m^3  winMaterialCp=glassCp J/(K*kg)  winAbsorptivity=glassAbsorptivity  winThermalK=glassThermalK W/(K*m)  winTransmissivity=glassTransmissivity  ventLength=0.1 m  ventHeight=0.1 m  extToWallHTC=htcExternal W/(K*m^2)  intToRoomHTC=htcInternal W/(K*m^2)  iniT=initialTemp K
      settings: InternalSimscapePortConfiguration="{\"Bottom\":[],\"Left\":[{\"id\":\"S\",\"label\":\"S\",\"type\":\"input\"},{\"id\":\"A\",\"label\":\"A\",\"type\":\"foundation.thermal.thermal\"}],\"Right\":[{\"id\":\"B\",\"label\":\"B\",\"type\":\"foundation.thermal.thermal\"}],\"Top\":[]}"
  Wall 2 : buildingEnergy_lib/Wall Selector  optWall=wallModelOption.wallSolarWin  wallLength=roomWidth m  wallHeight=roomHeight m  wallThickness=wallThickness m  wallMaterialDen=wallDensity kg/m^3  wallMaterialCp=wallCp J/(K*kg)  wallAbsorptivity=wallAbsorptivity  wallThermalK=wallThermalK W/(K*m)  winLength=roomWidth*windowFracWall2 m  winHeight=roomHeight m  winThickness=glassThickness m  winMaterialDen=glassDensity kg/m^3  winMaterialCp=glassCp J/(K*kg)  winAbsorptivity=glassAbsorptivity  winThermalK=glassThermalK W/(K*m)  winTransmissivity=glassTransmissivity  ventLength=0.1 m  ventHeight=0.1 m  extToWallHTC=htcExternal W/(K*m^2)  intToRoomHTC=htcInternal W/(K*m^2)  iniT=initialTemp K
      settings: InternalSimscapePortConfiguration="{\"Bottom\":[],\"Left\":[{\"id\":\"S\",\"label\":\"S\",\"type\":\"input\"},{\"id\":\"A\",\"label\":\"A\",\"type\":\"foundation.thermal.thermal\"}],\"Right\":[{\"id\":\"B\",\"label\":\"B\",\"type\":\"foundation.thermal.thermal\"}],\"Top\":[]}"
  Wall 3 : buildingEnergy_lib/Wall Selector  optWall=wallModelOption.wallSolarWin  wallLength=roomLength m  wallHeight=roomHeight m  wallThickness=wallThickness m  wallMaterialDen=wallDensity kg/m^3  wallMaterialCp=wallCp J/(K*kg)  wallAbsorptivity=wallAbsorptivity  wallThermalK=wallThermalK W/(K*m)  winLength=roomLength*windowFracWall3 m  winHeight=roomHeight m  winThickness=glassThickness m  winMaterialDen=glassDensity kg/m^3  winMaterialCp=glassCp J/(K*kg)  winAbsorptivity=glassAbsorptivity  winThermalK=glassThermalK W/(K*m)  winTransmissivity=glassTransmissivity  ventLength=0.1 m  ventHeight=0.1 m  extToWallHTC=htcExternal W/(K*m^2)  intToRoomHTC=htcInternal W/(K*m^2)  iniT=initialTemp K
      settings: InternalSimscapePortConfiguration="{\"Bottom\":[],\"Left\":[{\"id\":\"S\",\"label\":\"S\",\"type\":\"input\"},{\"id\":\"A\",\"label\":\"A\",\"type\":\"foundation.thermal.thermal\"}],\"Right\":[{\"id\":\"B\",\"label\":\"B\",\"type\":\"foundation.thermal.thermal\"}],\"Top\":[]}"
  Wall 4 : buildingEnergy_lib/Wall Selector  optWall=wallModelOption.wallSolarWin  wallLength=roomWidth m  wallHeight=roomHeight m  wallThickness=wallThickness m  wallMaterialDen=wallDensity kg/m^3  wallMaterialCp=wallCp J/(K*kg)  wallAbsorptivity=wallAbsorptivity  wallThermalK=wallThermalK W/(K*m)  winLength=roomWidth*windowFracWall4 m  winHeight=roomHeight m  winThickness=glassThickness m  winMaterialDen=glassDensity kg/m^3  winMaterialCp=glassCp J/(K*kg)  winAbsorptivity=glassAbsorptivity  winThermalK=glassThermalK W/(K*m)  winTransmissivity=glassTransmissivity  ventLength=0.1 m  ventHeight=0.1 m  extToWallHTC=htcExternal W/(K*m^2)  intToRoomHTC=htcInternal W/(K*m^2)  iniT=initialTemp K
      settings: InternalSimscapePortConfiguration="{\"Bottom\":[],\"Left\":[{\"id\":\"S\",\"label\":\"S\",\"type\":\"input\"},{\"id\":\"A\",\"label\":\"A\",\"type\":\"foundation.thermal.thermal\"}],\"Right\":[{\"id\":\"B\",\"label\":\"B\",\"type\":\"foundation.thermal.thermal\"}],\"Top\":[]}"
  Wall Thermal : PMIOPort  Side=Left
  Solar Radiation : PMIOPort  Port=2  Side=Left
  Qroom : PMIOPort  Port=3  Side=Left
  Data Center Heat : PMIOPort  Port=4  Side=Right
  Troom : PMIOPort  Port=5  Side=Right
  Grd : PMIOPort  Port=6  Side=Right
  connections:
  Qroom/RConn1 -- Room Volume/LConn1
  Floor/LConn1 -- Grd/RConn1
  Solar Radiation On Wall 2/RConn1 -- Wall 2/LConn1
  Wall 3/RConn1 -- Array Connection/LConn4
  Troom/RConn1 -- Room Volume/RConn1
  Solar Radiation On Wall 3/RConn1 -- Wall 3/LConn1
  Wall 1/RConn1 -- Array Connection/LConn2
  Convective Heat Transfer2/LConn1 -- Convective Heat Transfer4/LConn1 -- Convective Heat Transfer5/LConn1 -- Convective Heat Transfer3/LConn1 -- Wall Thermal/RConn1 -- Convective Heat Transfer1/LConn1
  Array Connection/RConn1 -- Room Volume/LConn2
  Solar Radiation/RConn1 -- Solar Radiation On Wall 1/LConn1 -- Solar Radiation On Wall 2/LConn1 -- Solar Radiation On Wall 4/LConn1 -- Solar Radiation On Wall 3/LConn1
  Wall 2/RConn1 -- Array Connection/LConn3
  Solar Radiation On Wall 1/RConn1 -- Wall 1/LConn1
  Room Volume/LConn3 -- Convective Heat Transfer/RConn1
  Floor/RConn1 -- Array Connection/LConn6
  Wall 4/RConn1 -- Array Connection/LConn5
  Solar Radiation On Wall 4/RConn1 -- Wall 4/LConn1
  Roof/RConn1 -- Array Connection/LConn1
  Convective Heat Transfer/LConn1 -- Data Center Heat/RConn1
  Convective Heat Transfer1/RConn1 -- Roof/LConn1
  Wall 1/LConn2 -- Convective Heat Transfer2/RConn1
  Wall 3/LConn2 -- Convective Heat Transfer3/RConn1
  Wall 2/LConn2 -- Convective Heat Transfer4/RConn1
  Wall 4/LConn2 -- Convective Heat Transfer5/RConn1
